simulink model "ex6_if_action2"  (R2021a)
settings: Solver=FixedStepAuto  StartTime=0.0  StopTime=10.0  FixedStep=1e-3  RelTol=1e-3
libraries: simulink x1
settings Model: Creator=reemb  LastModifiedBy=reemb

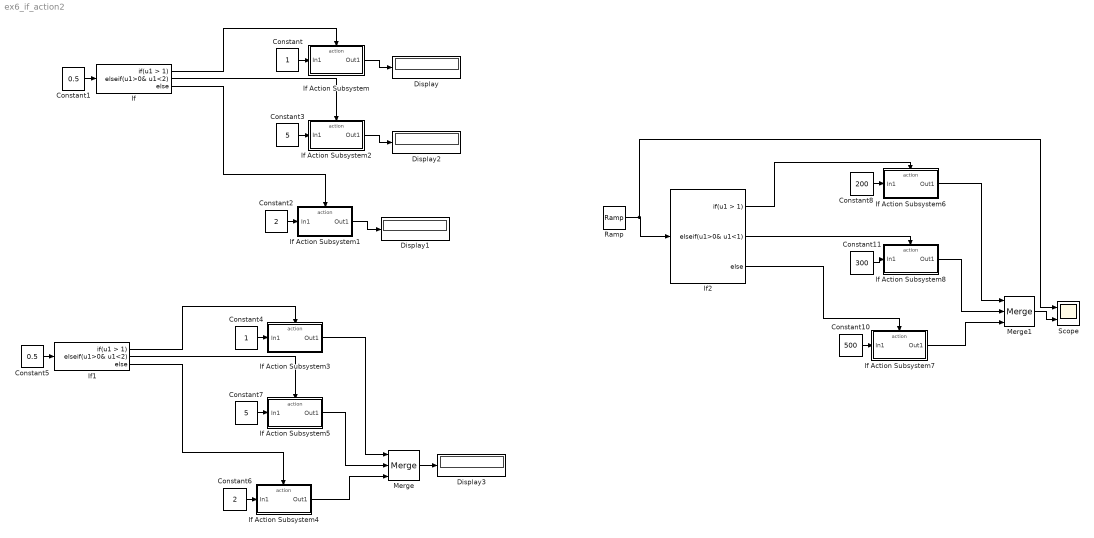
== system ex6_if_action2 ==
  Constant : Constant
  Constant1 : Constant  Value=0.5
  Constant10 : Constant  Value=500
  Constant11 : Constant  Value=300
  Constant2 : Constant  Value=2
  Constant3 : Constant  Value=5
  Constant4 : Constant
  Constant5 : Constant  Value=0.5
  Constant6 : Constant  Value=2
  Constant7 : Constant  Value=5
  Constant8 : Constant  Value=200
  Display{,1..3} (4 alike) : Display
  If : If  IfExpression=u1 > 1  ElseIfExpressions=u1>0& u1<2
  If Action Subsystem : Subsystem  TreatAsAtomicUnit=on
  If Action Subsystem1 : Subsystem  TreatAsAtomicUnit=on
  If Action Subsystem2 : Subsystem  TreatAsAtomicUnit=on
  If Action Subsystem3 : Subsystem  TreatAsAtomicUnit=on
  If Action Subsystem4 : Subsystem  TreatAsAtomicUnit=on
  If Action Subsystem5 : Subsystem  TreatAsAtomicUnit=on
  If Action Subsystem6 : Subsystem  TreatAsAtomicUnit=on
  If Action Subsystem7 : Subsystem  TreatAsAtomicUnit=on
  If Action Subsystem8 : Subsystem  TreatAsAtomicUnit=on
  If1 : If  IfExpression=u1 > 1  ElseIfExpressions=u1>0& u1<2
  If2 : If  IfExpression=u1 > 1  ElseIfExpressions=u1>0& u1<1
  Merge : Merge  Inputs=3
  Merge1 : Merge  Inputs=3
  Ramp : simulink/Sources/Ramp  slope=1  start=0  InitialOutput=-0.5
  Scope : Scope  NumInputPorts=2
  wires:
  If Action Subsystem/1(Out1) -> Display/1
  Constant/1 -> If Action Subsystem/1(In1)
  If/1 -> If Action Subsystem/Action
  Constant1/1 -> If/1
  Constant2/1 -> If Action Subsystem1/1(In1)
  If Action Subsystem1/1(Out1) -> Display1/1
  If/3 -> If Action Subsystem1/Action
  If Action Subsystem2/1(Out1) -> Display2/1
  Constant3/1 -> If Action Subsystem2/1(In1)
  If/2 -> If Action Subsystem2/Action
  If1/2 -> If Action Subsystem5/Action
  Constant7/1 -> If Action Subsystem5/1(In1)
  If Action Subsystem5/1(Out1) -> Merge/2
  If1/3 -> If Action Subsystem4/Action
  If Action Subsystem4/1(Out1) -> Merge/3
  Constant6/1 -> If Action Subsystem4/1(In1)
  Constant5/1 -> If1/1
  If1/1 -> If Action Subsystem3/Action
  Constant4/1 -> If Action Subsystem3/1(In1)
  If Action Subsystem3/1(Out1) -> Merge/1
  Merge/1 -> Display3/1
  Merge1/1 -> Scope/2
  If Action Subsystem6/1(Out1) -> Merge1/1
  Constant8/1 -> If Action Subsystem6/1(In1)
  If2/1 -> If Action Subsystem6/Action
  Ramp/1 -> Scope/1, If2/1
  Constant10/1 -> If Action Subsystem7/1(In1)
  If Action Subsystem7/1(Out1) -> Merge1/3
  If2/3 -> If Action Subsystem7/Action
  If Action Subsystem8/1(Out1) -> Merge1/2
  Constant11/1 -> If Action Subsystem8/1(In1)
  If2/2 -> If Action Subsystem8/Action

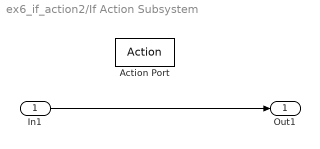
== system ex6_if_action2/If Action Subsystem ==
  In1 : Inport
  Action Port : ActionPort  ActionPortLabel=if(u1 > 1)
  Out1 : Outport
  wires:
  In1/1 -> Out1/1

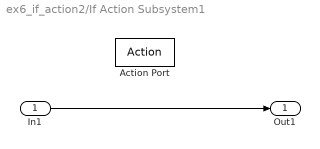
== system ex6_if_action2/If Action Subsystem1 ==
  In1 : Inport
  Action Port : ActionPort  ActionPortLabel=else
  Out1 : Outport
  wires:
  In1/1 -> Out1/1

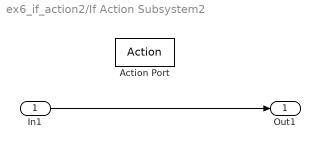
== system ex6_if_action2/If Action Subsystem2 ==
  In1 : Inport
  Action Port : ActionPort  ActionPortLabel=elseif( u1>0& u1<2)
  Out1 : Outport
  wires:
  In1/1 -> Out1/1

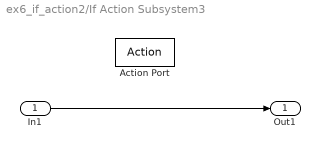
== system ex6_if_action2/If Action Subsystem3 ==
  In1 : Inport
  Action Port : ActionPort  ActionPortLabel=if(u1 > 1)
  Out1 : Outport
  wires:
  In1/1 -> Out1/1

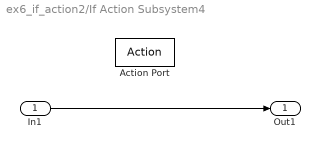
== system ex6_if_action2/If Action Subsystem4 ==
  In1 : Inport
  Action Port : ActionPort  ActionPortLabel=else
  Out1 : Outport
  wires:
  In1/1 -> Out1/1

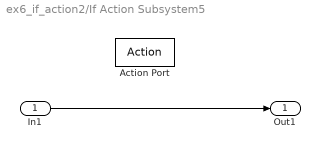
== system ex6_if_action2/If Action Subsystem5 ==
  In1 : Inport
  Action Port : ActionPort  ActionPortLabel=elseif( u1>0& u1<2)
  Out1 : Outport
  wires:
  In1/1 -> Out1/1

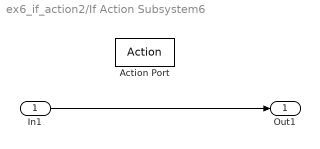
== system ex6_if_action2/If Action Subsystem6 ==
  In1 : Inport
  Action Port : ActionPort  ActionPortLabel=if(u1 > 1)
  Out1 : Outport
  wires:
  In1/1 -> Out1/1

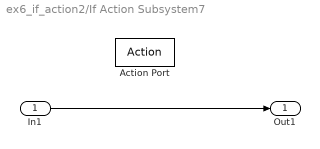
== system ex6_if_action2/If Action Subsystem7 ==
  In1 : Inport
  Action Port : ActionPort  ActionPortLabel=else
  Out1 : Outport
  wires:
  In1/1 -> Out1/1

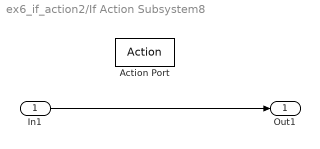
== system ex6_if_action2/If Action Subsystem8 ==
  In1 : Inport
  Action Port : ActionPort  ActionPortLabel=elseif( u1>0& u1<1)
  Out1 : Outport
  wires:
  In1/1 -> Out1/1
